simulink model "vrbounce"  (Simulink 7.4)
settings: Solver=ode45  SolverMode=SingleTasking  StartTime=0.0  StopTime=Inf  FixedStep=0.02  RelTol=1e-3
libraries: vrlib x2
Description:
  | Bouncing Ball
  | 
  | The vrbounce example visualizes a ball bouncing from a floor. The ball deforms as it hits
  | the floor keeping the volume of the ball constant. The deformation is achieved by
  | modifying the scale field of the ball.
settings Model: Creator=Straka  LastModifiedBy=Houska  CovMetricSettings=d  ExtModeTrigDuration=500
settings DataIOCC: LimitDataPoints=off  SaveOutput=off  SaveTime=off  SignalLoggingName=logsOut
settings OptimizationCC: BlockReduction=off  BooleanDataType=off  InlineInvariantSignals=on  InitFltsAndDblsToZero=on
settings DebuggingCC: CheckExecutionContextPreStartOutputMsg=on  CheckExecutionContextRuntimeOutputMsg=on  SignalResolutionControl=TryResolveAllWithWarning  SolverPrmCheckMsg=none  MultiTaskDSMMsg=warning  MultiTaskCondExecSysMsg=none  StrictBusMsg=None
settings HardwareCC: TargetUnknown=on
settings ModelReferenceCC: UpdateModelReferenceTargets=IfOutOfDate
settings SFSimCC: SimGenerateEmlReport=off
settings RTWCC: IncludeERTFirstTime=on
settings GRTTargetCC: TargetFcnLib=ansi_tfl_tmw.mat

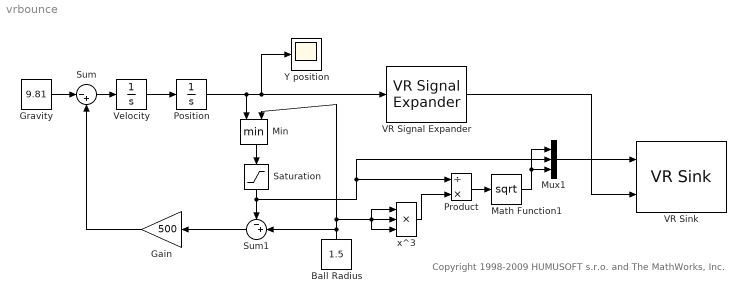
== system vrbounce ==
  note: Copyright 1998-2009 HUMUSOFT s.r.o. and The MathWorks, Inc.
  Ball Radius : Constant  Value=1.5  OutDataType=sfix(16)  OutScaling=2^0
  Gain : Gain  Gain=500  ParameterDataType=sfix(16)  ParameterScaling=2^0  OutDataType=sfix(16)  OutScaling=2^0  SaturateOnIntegerOverflow=on  OutDataTypeStr=Inherit: Same as input  ParamDataTypeStr=Inherit: Same as input
  Gravity : Constant  Value=9.81  OutDataType=sfix(16)  OutScaling=2^0
  Math Function1 : Math  Operator=sqrt  OutDataType=sfix(16)  OutScaling=2^0  SaturateOnIntegerOverflow=on
  Min : MinMax  Inputs=2  OutDataType=sfix(16)  OutScaling=2^0  ZeroCross=off  SaturateOnIntegerOverflow=on  InputSameDT=on
  Mux1 : Mux  Inputs=3
  Position : Integrator  InitialCondition=20  UpperSaturationLimit=Inf  LowerSaturationLimit=-Inf  ZeroCross=off
  Product : Product  Inputs=/*  OutDataType=sfix(16)  OutScaling=2^0  SaturateOnIntegerOverflow=on  InputSameDT=on  OutDataTypeStr=Inherit: Same as first input
  Saturation : Saturate  UpperLimit=Inf  LowerLimit=1e-4  ZeroCross=off  OutDataType=sfix(16)  OutScaling=2^0
  Sum : Sum  Inputs=|-+  OutDataType=sfix(16)  OutScaling=2^0  SaturateOnIntegerOverflow=on  InputSameDT=on  OutDataTypeStr=Inherit: Same as first input
  Sum1 : Sum  Inputs=-+|  OutDataType=sfix(16)  OutScaling=2^0  SaturateOnIntegerOverflow=on  InputSameDT=on  OutDataTypeStr=Inherit: Same as first input
  VR Signal Expander : vrlib/VR Signal Expander  SystemSampleTime=-1  outwidth=3  outidx=2
  VR Sink : vrlib/VR Sink  InstantiateOnLoad=on  SampleTime=0.02  ViewEnable=on  RemoteChange=off  RemoteView=off  FieldsWritten=Ball.scale.3.1.double#Ball.translation.3.1.double  WorldFileName=vrbounce.wrl  AutoView=on  VideoDimensions=[]  FigureProperties="{'Position', 'Name', 'Viewpoint', 'CameraBound', 'CameraDirection', 'CameraPosition', 'CameraUpVector', 'ZoomFactor', 'Antialiasing', 'Headlight', 'Lighting', 'NavPanel', 'StatusBar', 'ToolBar', 'Textures', 'Transparency', 'Wireframe', 'NavZones', 'NavMode', 'NavSpeed', 'Record2DCompressMethod', 'Record2DCompressQuality', 'Record2D', 'Record2DFileName', 'Record2DFPS'; [5.0000000000000000e+000  9.2000000000000000e+001  5.7600000000000000e+002  3.8000000000000000e+002], 'VR Bouncing Ball', 'Ball', 'on', [0.0000000000000000e+000  0.0000000000000000e+000 -1.0000000000000000e+000], [0.0000000000000000e+000  0.0000000000000000e+000  0.0000000000000000e+000], [0.0000000000000000e+000  1.0000000000000000e+000  0.0000000000000000e+000], [1.0000000000000000e+000], 'off', 'on', 'on', 'halfbar', 'off', 'on', 'on', 'on', 'off', 'off', 'examine', 'normal', 'auto', [7.5000000000000000e+001], 'off', '%f_anim_%n.avi', [1.5000000000000000e+001]}"
  Velocity : Integrator  UpperSaturationLimit=Inf  LowerSaturationLimit=-Inf  ZeroCross=off
  Y position : Scope
      settings: TimeRange=10  YMin=0  YMax=20
  x^3 : Product  Inputs=3  OutDataType=sfix(16)  OutScaling=2^0  SaturateOnIntegerOverflow=on  InputSameDT=on  OutDataTypeStr=Inherit: Same as first input
  wires:
  Velocity/1 -> Position/1
  Mux1/1 -> VR Sink/1
  VR Signal Expander/1 -> VR Sink/2
  Sum/1 -> Velocity/1
  Gravity/1 -> Sum/1
  Position/1 -> Y position/1, VR Signal Expander/1, Min/1
  Gain/1 -> Sum/2
  Min/1 -> Saturation/1
  Sum1/1 -> Gain/1
  Saturation/1 -> Sum1/1, Mux1/2, Product/1
  Product/1 -> Math Function1/1
  x^3/1 -> Product/2
  Math Function1/1 -> Mux1/1, Mux1/3
  Ball Radius/1 -> Sum1/2, Min/2, x^3/2, x^3/1, x^3/3
